simulink model "EPD629_WilliamsJ_AS04_P1_simulink"  (R2021b)
settings: Solver=VariableStepAuto  StartTime=0.0  StopTime=1  RelTol=1e-3
values from neighbouring files (symbols this model uses):
  A1 = -b/J    (= -20)    [EPD629_WilliamsJ_AS04.m]
  b = 0.001    [EPD629_WilliamsJ_AS04.m]
  B1 = 1/J    (= 20000)    [EPD629_WilliamsJ_AS04.m]
  C1 = 1    [EPD629_WilliamsJ_AS04.m]
  D1 = 0    [EPD629_WilliamsJ_AS04.m]
  J = 50e-6    (= 5e-05)    [EPD629_WilliamsJ_AS04.m]
  MotorTorque = 1    [EPD629_WilliamsJ_AS04.m]
settings Model: Creator=jwilli42  LastModifiedBy=jwilli42

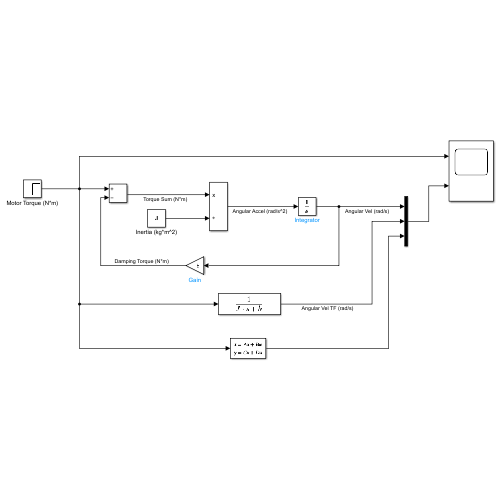
[thumbnail: Simulink's stored preview of the top-level diagram]
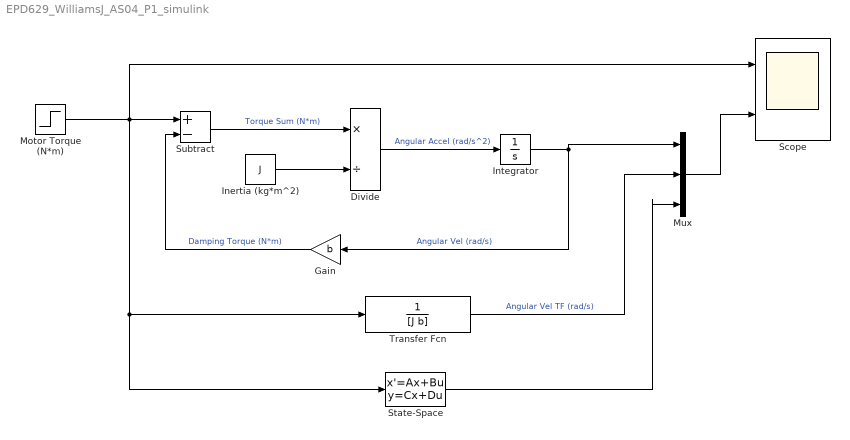
== system EPD629_WilliamsJ_AS04_P1_simulink ==
  Divide : Product  Inputs=*/
  Gain : Gain  Gain=b
  Inertia (kg*m^2) : Constant  Value=J
  Integrator : Integrator
  Motor Torque (N*m) : Step  Time=0  After=MotorTorque  SampleTime=0
  Mux : Mux  Inputs=3
  Scope : Scope  NumInputPorts=2
  State-Space : StateSpace  A=A1  B=B1  C=C1  D=D1  InitialCondition=0
  Subtract : Sum  Inputs=+-
  Transfer Fcn : TransferFcn  Denominator=[J b]
  wires:
  Motor Torque (N*m)/1 -> State-Space/1, Transfer Fcn/1, Scope/1, Subtract/1
  Subtract/1 -> Divide/1  "Torque Sum (N*m)"
  Divide/1 -> Integrator/1  "Angular Accel (rad/s^2)"
  Integrator/1 -> Gain/1, Mux/1  "Angular Vel (rad/s)"
  Inertia (kg*m^2)/1 -> Divide/2
  Gain/1 -> Subtract/2  "Damping Torque (N*m)"
  Mux/1 -> Scope/2
  Transfer Fcn/1 -> Mux/2  "Angular Vel TF (rad/s)"
  State-Space/1 -> Mux/3
